simulink model "CDPR_Test_Complete_Simulator_15_11"  (R2023b)
settings: Solver=VariableStepAuto  StartTime=0.0  StopTime=40  RelTol=1e-3
InitFcn:
  | run("CDPR_SIM_MAIN.m");
values from neighbouring files (symbols this model uses):
  a = [a1 a2 a3 a4]    [CDPR_SIM_MAIN.m]
  b = [b1 b1 b2 b2]    [CDPR_SIM_MAIN.m]
  G = m*[0; -9.81; 0]    [CDPR_SIM_MAIN.m]
  Jz = 1    [CDPR_SIM_MAIN.m]
  K_d = diag([8 8 1])    [CDPR_SIM_MAIN.m]
  K_i = diag([15 15 1])    [CDPR_SIM_MAIN.m]
  K_p = diag([10 10 1])    [CDPR_SIM_MAIN.m]
  m = 4    [CDPR_InverseKinematics_V2.m]    (also in CDPR_SIM_MAIN.m = 1; Kernel_translation_ELIAS_V2.m = length(A))
  y_ref = [0.5;0.5;0]    [CDPR_SIM_MAIN.m]
settings Model: Creator=magngrot  LastModifiedBy=magngrot
settings OptimizationCC: ReuseModelBlockBuffer=off

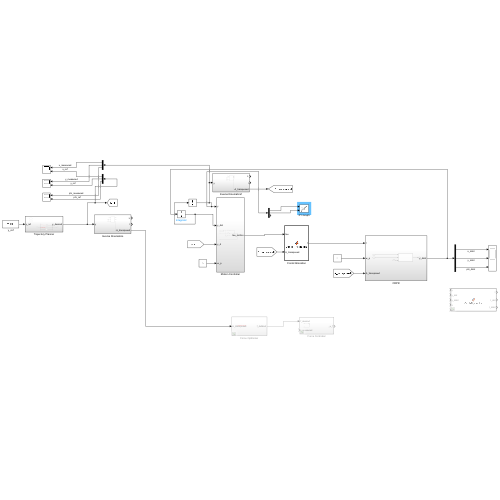
[thumbnail: Simulink's stored preview of the top-level diagram]
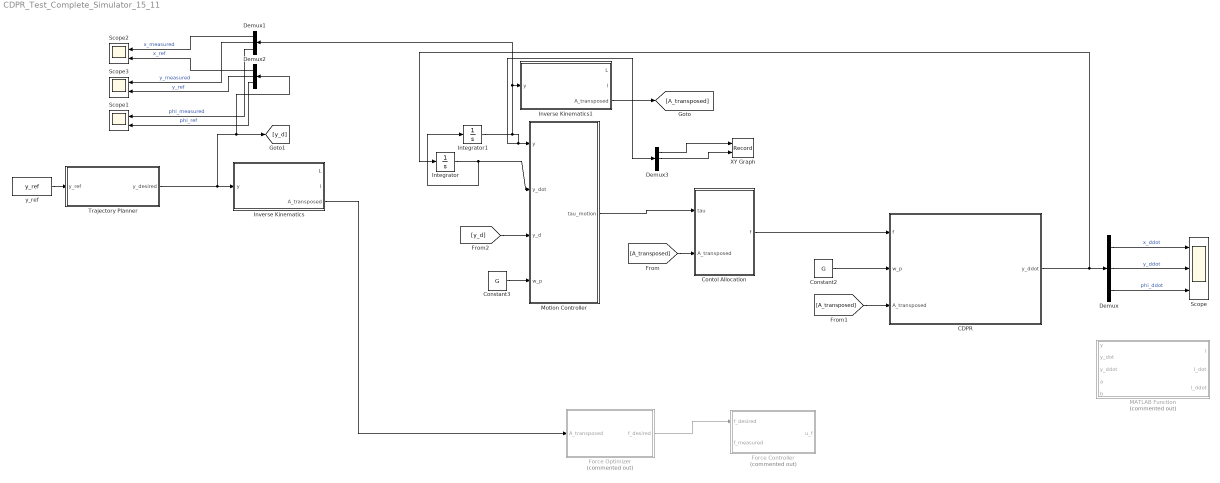
== system CDPR_Test_Complete_Simulator_15_11 ==
  CDPR : Subsystem
  Constant2 : Constant  Value=G
  Constant3 : Constant  Value=G
  Contol Allocation : MATLAB Function  TreatAsAtomicUnit=on
  Demux{,1..3} (4 alike) : Demux  Outputs=3
  Force Controller : Subsystem  Commented=on
  Force Optimizer : Subsystem  Commented=on
  Integrator : Integrator  InitialCondition=[0;0;0]
  Integrator1 : Integrator  InitialCondition=[0;0;0]
  Inverse Kinematics : Subsystem
  Inverse Kinematics1 : Subsystem
  MATLAB Function : MATLAB Function  Commented=on  TreatAsAtomicUnit=on
  Motion Controller : Subsystem
  Scope : Scope  NumInputPorts=3
  Scope1 : Scope  NumInputPorts=2
  Scope2 : Scope  NumInputPorts=2
  Scope3 : Scope  NumInputPorts=2
  Trajectory Planner : Subsystem
  XY Graph : Record  FileSettingsInternal="{\"entries\":[{\"content\":{\"excelSettings\":{\"content\":{},\"type\":\"Streamout.ExcelSettings\"}},\"type\":\"Streamout.FileSettingStorage\",\"uuid\":\"\"}],\"packageUris\":[\"http:\\/\\/schema.mathworks.com\\/mf0\\/streamout_blocks\\/R2020a\"],\"version\":\"1.0\"}"  Layout=[1 1]  SignalsInternal="{\"entries\":[{\"content\":{\"signals\":[{\"content\":{\"blockPath\":[],\"dimensions\":[1,1],\"domain\":\"\",\"lineColor\":\"#ff6929\",\"plots\":[1],\"port\":1,\"sid\":[\"\"],\"signalID\":53,\"signalName\":\"Demux3:1\"},\"type\":\"RecordBlkView.Signal\",\"uuid\":\"\"},{\"content\":{\"blockPath\":[],\"dimensions\":[1,1],\"domain\":\"\",\"lineColor\":\"#139fff\",\"plots\":[1],\"port\":2,\"sid\":[\"\"],\"signalID\":57,\"signalName\":\"Demux3:2\"},\"type\":\"RecordBlkView.Signal\",\"uuid\":\"\"}]},\"type\":\"RecordBlkView.InputSignals\",\"uuid\":\"\"}],\"packageUris\":[\"http:\\/\\/schema.mathworks.com\\/mf0\\/streamout_blocks\\/R2020a\"],\"version\":\"1.0\"}"  VisualizationBindings="{\"xyplotplugin\":{\"info\":[{\"series\":[{\"bindingParametersList\":[{\"parameter\":\"X-Axis\",\"signalID\":53,\"signalName\":\"Demux3:1\"},{\"parameter\":\"Y-Axis\",\"signalID\":57,\"signalName\":\"Demux3:2\"}],\"seriesID\":42676}],\"subplotID\":1}]}}"  CompatibilityTag=XY
  y_ref : Constant  Value=y_ref
  wires:
  Force Optimizer/1(f_desired) -> Force Controller/1(f_desired)
  y_ref/1 -> Trajectory Planner/1(y_ref)
  Trajectory Planner/1(y_desired) -> Inverse Kinematics/1(y), Demux2/1, [y_d]
  Motion Controller/1(tau_motion) -> Contol Allocation/1(tau)
  [A_transposed] -> Contol Allocation/2(A_transposed)
  Contol Allocation/1(f) -> CDPR/1(f)
  [A_transposed] -> CDPR/3(A_transposed)
  CDPR/1(y_ddot) -> Integrator/1, Demux/1
  [y_d] -> Motion Controller/3(y_d)
  Constant2/1 -> CDPR/2(w_p)
  Constant3/1 -> Motion Controller/4(w_p)
  Integrator/1 -> Motion Controller/2(y_dot), Integrator1/1
  Integrator1/1 -> Demux1/1, Inverse Kinematics1/1(y), Demux3/1, Motion Controller/1(y)
  Demux/1 -> Scope/1  "x_ddot"
  Demux/2 -> Scope/2  "y_ddot"
  Demux/3 -> Scope/3  "phi_ddot"
  Inverse Kinematics/3(A_transposed) -> Force Optimizer/1(A_transposed)
  Inverse Kinematics1/3(A_transposed) -> [A_transposed]
  Demux1/1 -> Scope2/1  "x_measured"
  Demux2/1 -> Scope2/2  "x_ref"
  Demux1/2 -> Scope3/1  "y_measured"
  Demux2/2 -> Scope3/2  "y_ref"
  Demux1/3 -> Scope1/1  "phi_measured"
  Demux2/3 -> Scope1/2  "phi_ref"
  Demux3/1 -> XY Graph/1
  Demux3/2 -> XY Graph/2

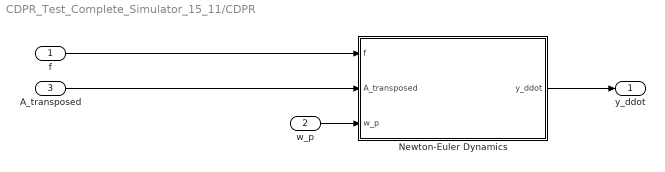
== system CDPR_Test_Complete_Simulator_15_11/CDPR ==
  f : Inport
  w_p : Inport  Port=2
  A_transposed : Inport  Port=3
  "Newton-Euler Dynamics " : Subsystem
  y_ddot : Outport
  wires:
  "Newton-Euler Dynamics "/1(y_ddot) -> y_ddot/1
  A_transposed/1 -> "Newton-Euler Dynamics "/2(A_transposed)
  f/1 -> "Newton-Euler Dynamics "/1(f)
  w_p/1 -> "Newton-Euler Dynamics "/3(w_p)

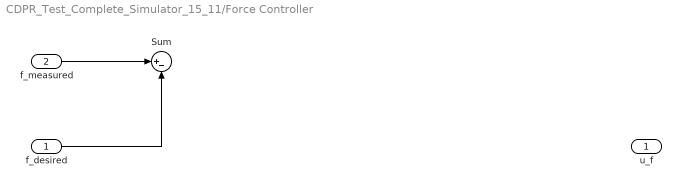
== system CDPR_Test_Complete_Simulator_15_11/Force Controller ==
  f_desired : Inport
  f_measured : Inport  Port=2
  Sum : Sum  Inputs=|+-
  u_f : Outport
  wires:
  f_measured/1 -> Sum/1
  f_desired/1 -> Sum/2

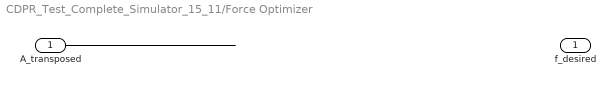
== system CDPR_Test_Complete_Simulator_15_11/Force Optimizer ==
  A_transposed : Inport
  f_desired : Outport
  wires:
  A_transposed/1 -> ?

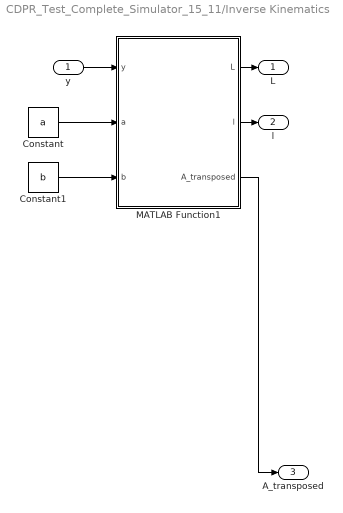
== system CDPR_Test_Complete_Simulator_15_11/Inverse Kinematics ==
  y : Inport
  Constant : Constant  Value=a
  Constant1 : Constant  Value=b
  MATLAB Function1 : MATLAB Function  TreatAsAtomicUnit=on
  L : Outport
  l : Outport  Port=2
  A_transposed : Outport  Port=3
  wires:
  Constant/1 -> MATLAB Function1/2(a)
  MATLAB Function1/3(A_transposed) -> A_transposed/1
  Constant1/1 -> MATLAB Function1/3(b)
  y/1 -> MATLAB Function1/1(y)
  MATLAB Function1/1(L) -> L/1
  MATLAB Function1/2(l) -> l/1

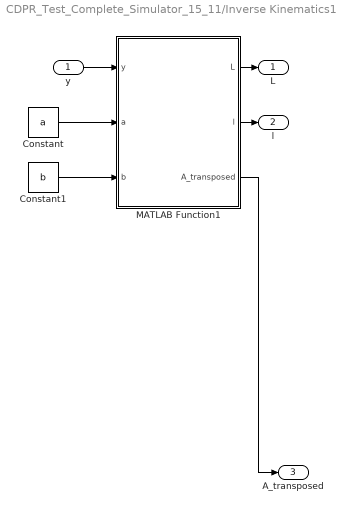
== system CDPR_Test_Complete_Simulator_15_11/Inverse Kinematics1 ==
  y : Inport
  Constant : Constant  Value=a
  Constant1 : Constant  Value=b
  MATLAB Function1 : MATLAB Function  TreatAsAtomicUnit=on
  L : Outport
  l : Outport  Port=2
  A_transposed : Outport  Port=3
  wires:
  Constant/1 -> MATLAB Function1/2(a)
  MATLAB Function1/3(A_transposed) -> A_transposed/1
  Constant1/1 -> MATLAB Function1/3(b)
  y/1 -> MATLAB Function1/1(y)
  MATLAB Function1/1(L) -> L/1
  MATLAB Function1/2(l) -> l/1

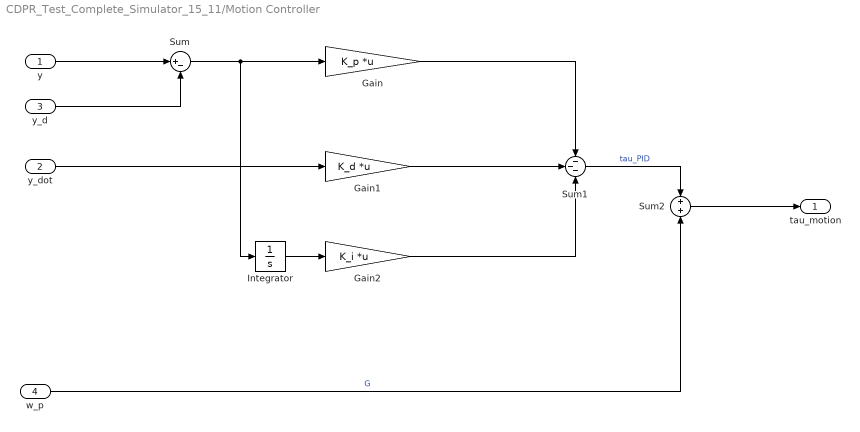
== system CDPR_Test_Complete_Simulator_15_11/Motion Controller ==
  y : Inport
  y_dot : Inport  Port=2
  y_d : Inport  Port=3
  w_p : Inport  Port=4
  Gain : Gain  Gain=K_p  Multiplication=Matrix(K*u)
  Gain1 : Gain  Gain=K_d  Multiplication=Matrix(K*u)
  Gain2 : Gain  Gain=K_i  Multiplication=Matrix(K*u)
  Integrator : Integrator
  Sum : Sum  Inputs=|+-
  Sum1 : Sum  Inputs=---
  Sum2 : Sum  Inputs=+|+
  tau_motion : Outport
  wires:
  y/1 -> Sum/1
  y_d/1 -> Sum/2
  Sum/1 -> Integrator/1, Gain/1
  y_dot/1 -> Gain1/1
  Sum2/1 -> tau_motion/1
  w_p/1 -> Sum2/2  "G"
  Gain1/1 -> Sum1/2
  Gain/1 -> Sum1/1
  Integrator/1 -> Gain2/1
  Gain2/1 -> Sum1/3
  Sum1/1 -> Sum2/1  "tau_PID"

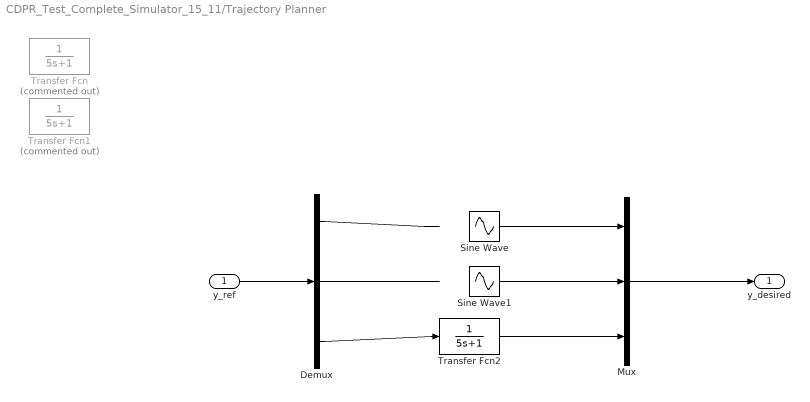
== system CDPR_Test_Complete_Simulator_15_11/Trajectory Planner ==
  y_ref : Inport
  Demux : Demux  Outputs=3
  Mux : Mux  Inputs=3
  Sine Wave : Sin  Amplitude=0.5  Frequency=0.5  Phase=pi/2  SampleTime=0
  Sine Wave1 : Sin  Amplitude=0.5  Frequency=0.5  SampleTime=0
  Transfer Fcn : TransferFcn  Commented=on  Denominator=[5 1]
  Transfer Fcn1 : TransferFcn  Commented=on  Denominator=[5 1]
  Transfer Fcn2 : TransferFcn  Denominator=[5 1]
  y_desired : Outport
  wires:
  y_ref/1 -> Demux/1
  Demux/1 -> ?
  Demux/2 -> ?
  Demux/3 -> Transfer Fcn2/1
  Sine Wave/1 -> Mux/1
  Sine Wave1/1 -> Mux/2
  Transfer Fcn2/1 -> Mux/3
  Mux/1 -> y_desired/1

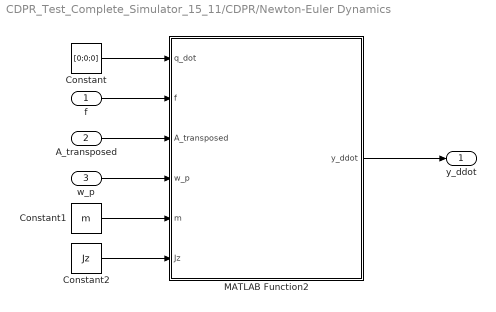
== system CDPR_Test_Complete_Simulator_15_11/CDPR/Newton-Euler Dynamics  ==
  f : Inport
  A_transposed : Inport  Port=2
  w_p : Inport  Port=3
  Constant : Constant  Value=[0;0;0]
  Constant1 : Constant  Value=m
  Constant2 : Constant  Value=Jz
  MATLAB Function2 : MATLAB Function  TreatAsAtomicUnit=on
  y_ddot : Outport
  wires:
  MATLAB Function2/1(y_ddot) -> y_ddot/1
  f/1 -> MATLAB Function2/2(f)
  Constant/1 -> MATLAB Function2/1(q_dot)
  A_transposed/1 -> MATLAB Function2/3(A_transposed)
  Constant1/1 -> MATLAB Function2/5(m)
  Constant2/1 -> MATLAB Function2/6(Jz)
  w_p/1 -> MATLAB Function2/4(w_p)

== matlab function CDPR_Test_Complete_Simulator_15_11/Inverse Kinematics/MATLAB Function1 ==
  data: y input; L output; a input; b input; l output; A_transposed output
function [L,l,A_transposed] = InverseKinematics(y,a,b)

[L,l,A_transposed] = CDPR_InverseKinematics_V2(y, a, b);

== matlab function CDPR_Test_Complete_Simulator_15_11/MATLAB Function ==
  data: y input; l output; y_dot input; y_ddot input; a input; b input; l_dot output; l_ddot output
function [l,l_dot,l_ddot] = CableDynamics(y, y_dot, y_ddot, a, b)
[l,l_dot,l_ddot] = CableDynamics(y, y_dot, y_ddot, a, b);

== matlab function CDPR_Test_Complete_Simulator_15_11/Inverse Kinematics1/MATLAB Function1 ==
  data: y input; L output; a input; b input; l output; A_transposed output
function [L,l,A_transposed] = InverseKinematics(y,a,b)

[L,l,A_transposed] = CDPR_InverseKinematics_V2(y, a, b);

== matlab function CDPR_Test_Complete_Simulator_15_11/Contol Allocation ==
  data: tau input; f output; A_transposed input
function f = Control_Allocation(tau, A_transposed)

f = CDPR_Control_Allocation(tau, A_transposed);
end

== matlab function CDPR_Test_Complete_Simulator_15_11/CDPR/Newton-Euler Dynamics /MATLAB Function2 ==
  data: q_dot input; y_ddot output; f input; A_transposed input; w_p input; m input; Jz input
function y_ddot = NewtonEuler_Dynamics(q_dot, f, A_transposed, w_p, m, Jz)

y_ddot = CDPR_NewtonEuler_Dynamics(q_dot, f, A_transposed, w_p, m, Jz);
